simulink model "flight_simulator"  (R2022a)
settings: Solver=VariableStepAuto  StartTime=0.0  StopTime=10.0  RelTol=1e-3
libraries: aerolibwind2 x2, aerolibatmos2 x1, shared6dof x1
settings Model: Creator=usmaanyaqoob  LastModifiedBy=usmaanyaqoob

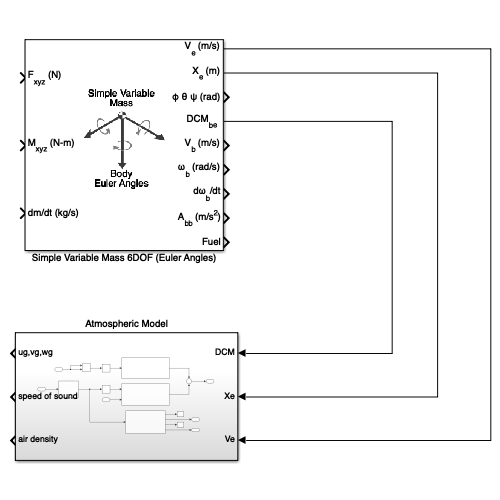
[thumbnail: Simulink's stored preview of the top-level diagram]
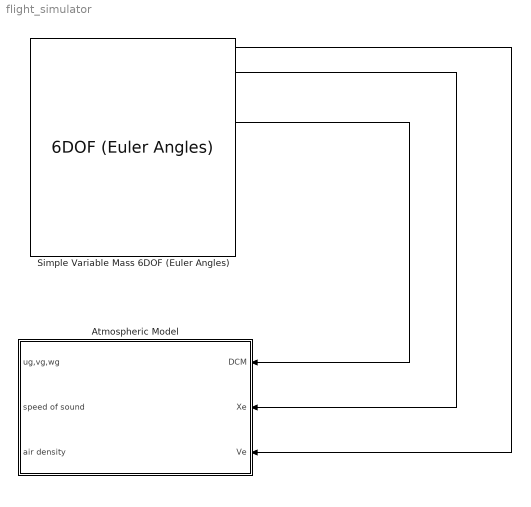
== system flight_simulator ==
  Atmospheric Model : Subsystem
  Simple Variable Mass 6DOF (Euler Angles) : shared6dof/6DOF (Euler Angles)  units=Metric (MKS)  mtype=Simple Variable  rep=Euler Angles  xme_0=[0 0 0]  Vm_0=[0 0 0]  eul_0=[0 0 0]  pm_0=[0 0 0]  mass_0=1.0  mass_e=0.5  mass_f=2.0  inertia=eye(3)  inertia_e=eye(3)  inertia_f=2*eye(3)  k_quat=1.0  vre_flag=off  abi_flag=off  aMode=0  xme_statename=''  Vm_statename=''  eul_statename=''  quat_statename=''  pm_statename=''  mass_statename=''
      settings: SourceProductBaseCode=AE,PW,DR,MT,VE
  wires:
  Simple Variable Mass 6DOF (Euler Angles)/4 -> Atmospheric Model/1(DCM)
  Simple Variable Mass 6DOF (Euler Angles)/2 -> Atmospheric Model/2(Xe)
  Simple Variable Mass 6DOF (Euler Angles)/1 -> Atmospheric Model/3(Ve)

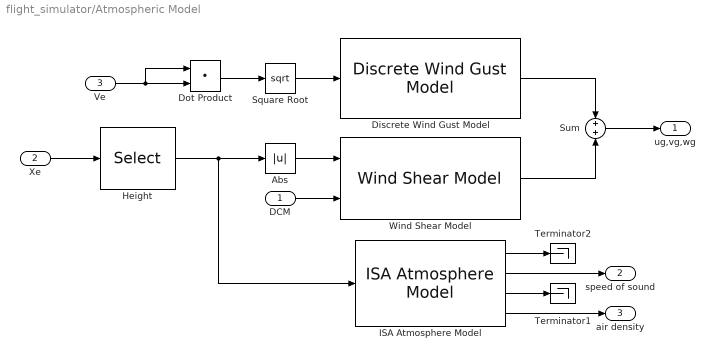
== system flight_simulator/Atmospheric Model ==
  DCM : Inport
  Xe : Inport  Port=2
  Ve : Inport  Port=3
  Abs : Abs  SaturateOnIntegerOverflow=off
  Discrete Wind Gust Model : aerolibwind2/Discrete Wind Gust Model  units=Metric (MKS)  Gx=on  Gy=on  Gz=on  t_0=5  d_m=[120 120 80]  v_m=[3.5 3.5 3.0]
  Dot Product : DotProduct  OutDataTypeStr=Inherit: Inherit via internal rule
  Height : Selector  InputPortWidth=3  IndexOptions=Index vector (dialog)  Indices=[3]  OutputSizes=1
  ISA Atmosphere Model : aerolibatmos2/ISA Atmosphere Model  custom=off  g=9.80665  gamma=1.4  R=287.0531  L=0.0065  h_trop=11000  h_strat=20000  rho0=1.225  P0=101325  T0=288.15  h0=0
  Square Root : Sqrt
  Sum : Sum
  Terminator1 : Terminator
  Terminator2 : Terminator
  Wind Shear Model : aerolibwind2/Wind Shear Model  units=Metric (MKS)  phase=Category C - Terminal Flight Phase  W_20=15  Wdeg=0
  ug,vg,wg : Outport
  speed of sound : Outport  Port=2
  air density : Outport  Port=3
  wires:
  Xe/1 -> Height/1
  Height/1 -> Abs/1, ISA Atmosphere Model/1
  DCM/1 -> Wind Shear Model/2
  Ve/1 -> Dot Product/1, Dot Product/2
  Dot Product/1 -> Square Root/1
  Square Root/1 -> Discrete Wind Gust Model/1
  Discrete Wind Gust Model/1 -> Sum/1
  Wind Shear Model/1 -> Sum/2
  Abs/1 -> Wind Shear Model/1
  Sum/1 -> ug,vg,wg/1
  ISA Atmosphere Model/2 -> speed of sound/1
  ISA Atmosphere Model/4 -> air density/1
  ISA Atmosphere Model/3 -> Terminator1/1
  ISA Atmosphere Model/1 -> Terminator2/1
